simulink model "smpld_data_sys_"  (R2025b)
settings: Solver=ode45  StartTime=0.0  StopTime=20  FixedStep=T  MaxStep=0.01  RelTol=1e-12  AbsTol=1e-12  EnableMultiTasking=on
values from neighbouring files (symbols this model uses):
  T = 0.2764    [lab3.m]
libraries: cstblocks x2
settings Model: Creator=cnielsen  LastModifiedBy=hasan_khan
settings SolverCC: AutoScaleAbsTol=off  AlgebraicLoopSolver=TrustRegion
settings DataIOCC: SaveFormat=Array  SignalLoggingSaveFormat=ModelDataLogs  SaveOutput=off  SaveTime=off  ReturnWorkspaceOutputs=off  Refine=5
settings OptimizationCC: ExpressionDepthLimit=2147483647.0  LifeSpan=inf
settings DebuggingCC: UnderspecifiedInitializationDetection=Classic  MergeDetectMultiDrivingBlocksExec=none  SolverPrmCheckMsg=warning  FcnCallInpInsideContextMsg=warning  UnconnectedInputMsg=warning  UnconnectedOutputMsg=warning  UnconnectedLineMsg=warning  StateNameClashWarn=warning  SFUnexpectedBacktrackingDiag=warning  SFNoUnconditionalDefaultTransitionDiag=warning  SFExecutionAtInitializationDiag=none  ArithmeticOperatorsInVariantConditions=warning
settings HardwareCC: ProdBitPerPointer=32.0  ProdBitPerSizeT=32.0  ProdBitPerPtrDiffT=32.0  ProdLargestAtomicFloat=None  ProdIntDivRoundTo=Undefined  ProdEndianess=Unspecified  ProdWordSize=32.0  ProdHWDeviceType=32-bit Generic
settings ModelReferenceCC: PropagateSignalLabelsOutOfModel=off
settings SFSimCC: SimUseLocalCustomCode=off  CustomCodeUndefinedFunction=UseInterfaceOnly
settings RTWCC: RTWUseLocalCustomCode=off  GPUComputeCapability=3.5
settings CodeAppCC: StateflowObjectComments=on
settings GRTTargetCC: TargetLangStandard=C89/C90 (ANSI)  CombineOutputUpdateFcns=off  GRTInterface=on
settings ConfigComp: CovMetricSettings=dw  CovSaveCumulativeToWorkspaceVar=on  CovSaveSingleToWorkspaceVar=on  CovExternalEMLEnable=off
settings SimscapeCC: SimscapeLogDecimation=1  SimscapeLogDataHistory=5000

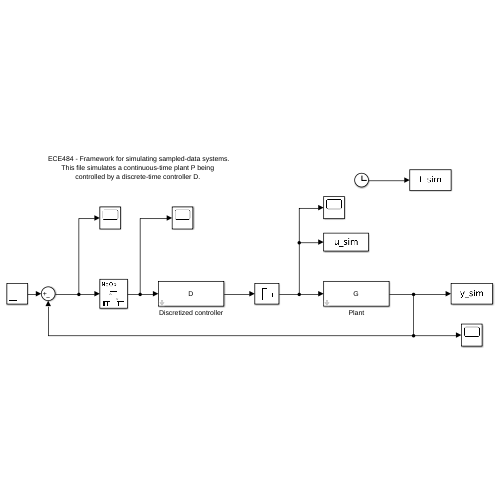
[thumbnail: Simulink's stored preview of the top-level diagram]
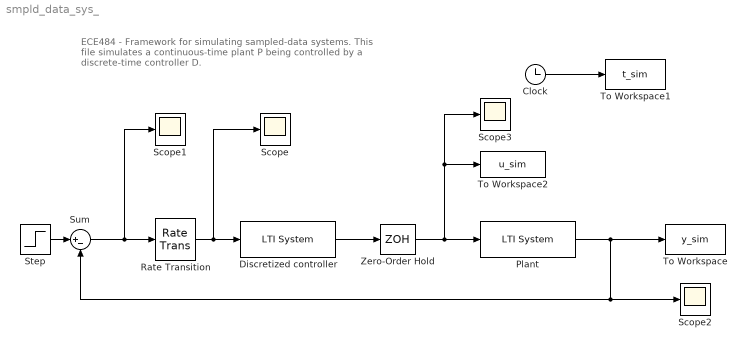
== system smpld_data_sys_ ==
  note: ECE484 - Framework for simulating sampled-data systems.
      | This file simulates a continuous-time plant P being
      | controlled by a discrete-time controller D.
  Clock : Clock
  Discretized controller : cstblocks/LTI System  sys=D  IC=[]  PadeOrder=0
  Plant : cstblocks/LTI System  sys=G  IC=[]  PadeOrder=0
  Rate Transition : RateTransition  OutPortSampleTime=T
  Scope{,1..3} (4 alike) : Scope
      Scope settings: TimeSpan=auto  ActiveDisplayYMinimum=-7.94103  ActiveDisplayYMaximum=8.76404
      Scope1 settings: TimeSpan=auto  ActiveDisplayYMinimum=-7.94103  ActiveDisplayYMaximum=8.76404
      Scope2 settings: TimeSpan=auto  ActiveDisplayYMinimum=0.57881075934071813  ActiveDisplayYMaximum=1.1841181311679858  DataLoggingVariableName=ScopeData2
      Scope3 settings: TimeSpan=auto  ActiveDisplayYMinimum=-5.837808682573888  ActiveDisplayYMaximum=5.0007716318251436
  Step : Step  Time=0  SampleTime=0.2764
  Sum : Sum  Inputs=|+-
  To Workspace : ToWorkspace  VariableName=y_sim  SampleTime=-1
  To Workspace1 : ToWorkspace  VariableName=t_sim  SampleTime=-1
  To Workspace2 : ToWorkspace  VariableName=u_sim
  Zero-Order Hold : ZeroOrderHold  SampleTime=T
  wires:
  Clock/1 -> To Workspace1/1
  Discretized controller/1 -> Zero-Order Hold/1
  Step/1 -> Sum/1
  Plant/1 -> To Workspace/1, Sum/2, Scope2/1
  Sum/1 -> Rate Transition/1, Scope1/1
  Zero-Order Hold/1 -> Plant/1, To Workspace2/1, Scope3/1
  Rate Transition/1 -> Discretized controller/1, Scope/1
